simulink model "nadir_pointing_magnetorquers"  (R2021a)
settings: Solver=VariableStepAuto  StartTime=0.0  StopTime=Torb  RelTol=1e-3
libraries: sharedtransform x2
settings Model: Creator=Laura  LastModifiedBy=Laura

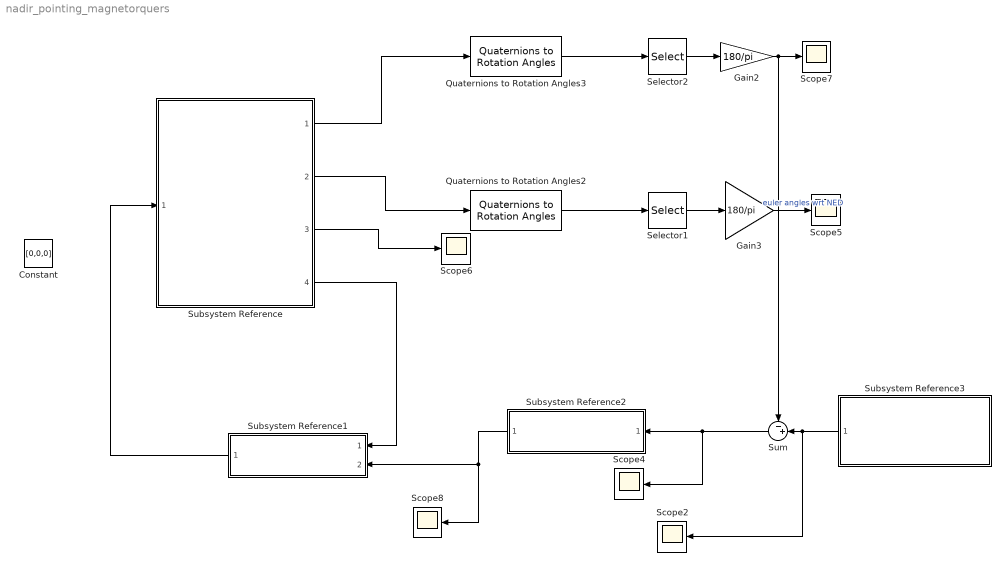
== system nadir_pointing_magnetorquers ==
  Constant : Constant  Value=[0,0,0]
  Gain2 : Gain  Gain=180/pi
  Gain3 : Gain  Gain=180/pi
  Quaternions to Rotation Angles2 : sharedtransform/Quaternions to Rotation Angles  rotationOrder=ZYX  aMode=aMode
      settings: SourceProductBaseCode=AE,PW,DR,MT,UV,VE
  Quaternions to Rotation Angles3 : sharedtransform/Quaternions to Rotation Angles  rotationOrder=ZYX  aMode=aMode
      settings: SourceProductBaseCode=AE,PW,DR,MT,UV,VE
  Scope{2,4..8} (6 alike) : Scope
  Selector1 : Selector  InputPortWidth=3  IndexOptions=Index vector (dialog)  Indices=[3 2 1]  OutputSizes=1
  Selector2 : Selector  InputPortWidth=3  IndexOptions=Index vector (dialog)  Indices=[3 2 1]  OutputSizes=1
  Subsystem Reference : Subsystem  ReferencedSubsystem=DKE_nadirpointing_magneto
  Subsystem Reference1 : Subsystem  ReferencedSubsystem=PID_nadir
  Subsystem Reference2 : Subsystem  ReferencedSubsystem=PID
  Subsystem Reference3 : Subsystem  ReferencedSubsystem=ThreeAxesSignals
  Sum : Sum  Inputs=-+|
  wires:
  Selector2/1 -> Gain2/1
  Quaternions to Rotation Angles3/1 -> Selector2/1
  Subsystem Reference/1 -> Quaternions to Rotation Angles3/1
  Subsystem Reference2/1 -> Subsystem Reference1/2, Scope8/1
  Subsystem Reference3/1 -> Scope2/1, Sum/2
  Selector1/1 -> Gain3/1
  Sum/1 -> Scope4/1, Subsystem Reference2/1
  Subsystem Reference/3 -> Scope6/1
  Gain3/1 -> Scope5/1  "euler angles wrt NED"
  Subsystem Reference1/1 -> Subsystem Reference/1
  Quaternions to Rotation Angles2/1 -> Selector1/1
  Gain2/1 -> Sum/1, Scope7/1
  Subsystem Reference/2 -> Quaternions to Rotation Angles2/1
  Subsystem Reference/4 -> Subsystem Reference1/1
